simulink model "TECMD_OptimisationTemplate"  (R2021a)
settings: Solver=daessc  StartTime=0.0  StopTime=7192.4000005722046  FixedStep=1  MaxStep=1  RelTol=1e-3  AbsTol=1e-3
libraries: fl_lib x7, nesl_utility x7, BatteryLibrary_lib x1
settings Model: Creator=widana_d  LastModifiedBy=widana_d
settings SolverCC: AutoScaleAbsTol=off  AlgebraicLoopSolver=TrustRegion
settings DataIOCC: ExternalInput=currData  LoadExternalInput=on  SaveState=on  ReturnWorkspaceOutputsName=SDOSimTest_Log
settings DebuggingCC: SymbolicDimsDataTypeCodeGenerationDiagnostic=none  SFMachineParentedDataDiag=warning
settings SFSimCC: CustomCodeUndefinedFunction=UseInterfaceOnly
settings SimscapeCC: SimscapeLogType=all  SimscapeLogSimulationStatistics=on  SimscapeLogDataHistory=10000

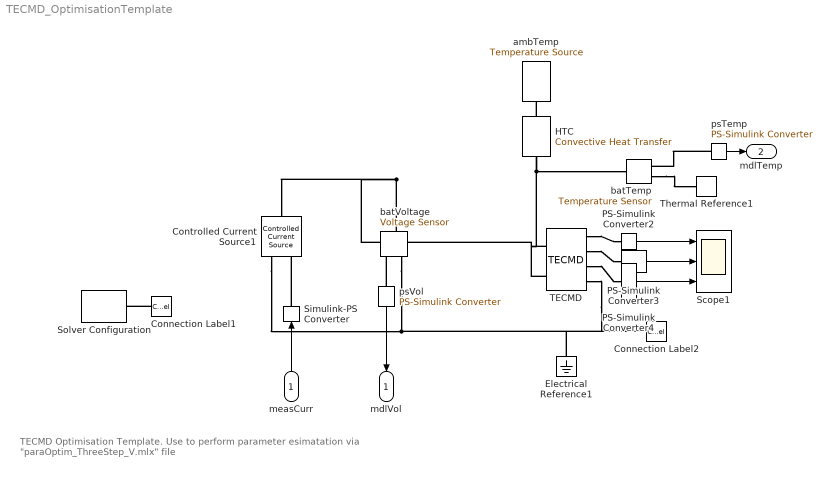
== system TECMD_OptimisationTemplate ==
  note: TECMD Optimisation Template.
      | Use to perform parameter esimatation via "paraOptim_ThreeStep_V.mlx" file
  measCurr : Inport
  Connection Label1 : ConnectionLabel  Label=solver
  Connection Label2 : ConnectionLabel  Label=solver
  Controlled Current Source1 : fl_lib/Electrical/Electrical Sources/Controlled Current Source
  Electrical Reference1 : fl_lib/Electrical/Electrical Elements/Electrical Reference
  HTC : fl_lib/Thermal/Thermal Elements/Convective Heat Transfer  area=cellArea m^2  heat_tr_coeff=h W/(m^2 * K)  T_specify=off  T_priority=None  T=0 K  T_nominal_specify=off  T_nominal_unit=K  T_nominal_value=1  Q_specify=off  Q_priority=None  Q=0 W  Q_nominal_specify=off  Q_nominal_unit=W  Q_nominal_value=1
  PS-Simulink Converter2 : nesl_utility/PS-Simulink Converter  PhysicalDomain=network_engine_domain  SubClassName=ps_output  LeftPortType=input  RightPortType=output  PseudoPeriodic=off  Frequencies=[]  Unit=inherit  AffineConversion=off
      settings: SourceProductBaseCode=PW,SS
  PS-Simulink Converter3 : nesl_utility/PS-Simulink Converter  PhysicalDomain=network_engine_domain  SubClassName=ps_output  LeftPortType=input  RightPortType=output  PseudoPeriodic=off  Frequencies=[]  Unit=inherit  AffineConversion=off
      settings: SourceProductBaseCode=PW,SS
  PS-Simulink Converter4 : nesl_utility/PS-Simulink Converter  PhysicalDomain=network_engine_domain  SubClassName=ps_output  LeftPortType=input  RightPortType=output  PseudoPeriodic=off  Frequencies=[]  Unit=inherit  AffineConversion=off
      settings: SourceProductBaseCode=PW,SS
  Scope1 : Scope  NumInputPorts=3
  Simulink-PS Converter : nesl_utility/Simulink-PS Converter  PhysicalDomain=network_engine_domain  SubClassName=ps_input  LeftPortType=input  RightPortType=output  PseudoPeriodic=off  Frequencies=[]  NoiseDistribution=none  NoiseParameters=[]  Unit=1  AffineConversion=off  FilteringAndDerivatives=provide  SimscapeFilterOrder=1  InputFilterTimeConstant=0.001  UdotUserProvided=0
      settings: SourceProductBaseCode=PW,SS
  Solver Configuration : nesl_utility/Solver Configuration  PhysicalDomain=network_engine_domain  SubClassName=solver  LeftPortType=input  RightPortType=generic  Tones=[]  Harmonics=[]  SimulateNoise=off  Profile=off  UseLocalSampling=off  EnableSwitchedLinearOptims=on  FrequencyDomain=off  UseCCode=off  RelTol=0.001  AbsTol=1e-06  MinStep=1e-09  ToWorkspace=off  RevertToSquareIcSolve=off  NumHomotopyIterations=100  PhasorMode=off  PhasorModeNumHarmonics=1  DoDC=off  ResidualTolerance=1e-09  UseLocalSolver=off  LocalSolverChoice=NE_BACKWARD_EULER_ADVANCER  LocalSolverSampleTime=0.001  DoFixedCost=off  MaxNonlinIter=3  MaxModeIter=2  ComputeImpulses=off  ImpulseIterations=2  LinearAlgebra=auto  EquationFormulation=NE_TIME_EF  DelaysMemoryBudget=1024  AutomaticFiltering=on  FilteringTimeConstant=0.001  PartitionStorageMethod=AS_NEEDED  PartitionMemoryBudget=1024  PartitionMethod=ROBUST
      settings: SourceProductName=Utilities
  TECMD : BatteryLibrary_lib/Models/TECMD  RoRef=RoRef Ohm  RpRef=RpRef Ohm  TaupRef=TaupRef s  TauRef=TauRef s  Cn=Cn hr*A  z0=z0  Cp=Cp J/K  Tref=Tref K  Ea_Ro=Ea_Ro kJ/mol  Ea_Rp=Ea_Rp kJ/mol  Ea_Taup=Ea_Taup kJ/mol  Ea_Tau=Ea_Tau kJ/mol  T0=T0 K  refSoC=[0 : 100]' / 100  refOCV=[2.8593, 2.9274, 2.9956, 3.061969, 3.1232121621911, 3.15470394885229, 3.18512081795661, 3.21447466451004, 3.23983418251859, 3.25947590964635, 3.27879990917066, 3.29791977833839, 3.31626752560394, 3.33307563518842, 3.34970466285667, 3.36646662161759, 3.38398642592777, 3.39826374829121, 3.41202994917722, 3.4257108806197, 3.43855191633442, 3.45201772552158, 3.46575676444741, 3.47936243182409, 3.49084733247506, 3.50171432332238, 3.51269575981572, 3.52363960685895, 3.5336162322311, 3.54266659043136, 3.55146484401725, 3.56028882406785, 3.57078460389872, 3.58129525123674, 3.59144125445442, 3.60158725767211, 3.6115458412695, 3.62096628333315, 3.63026578569043, 3.63956528804771, 3.64823659910672, 3.65653982870753, 3.66499745309439, 3.67345507748124, 3.68147228638747, 3.68961276847631, 3.69798562783594, 3.70635848719557, 3.71487037672799, 3.72380783932121, 3.73289437418429, 3.74198090904738, 3.75102505534397, 3.76031929016191, 3.76983942070008, 3.77935955123825, 3.78884224697143, 3.79882047635899, 3.80921579355511, 3.81961111075122, 3.83069866787416, 3.84218843373057, 3.85281884527956, 3.86344925682856, 3.873689991993, 3.8823694410751, 3.89044668294659, 3.89852392481808, 3.90617127176311, 3.91300386552967, 3.92012910853992, 3.92725435155017, 3.93469242351412, 3.94356346975952, 3.95323912490892, 3.96292857788519, 3.97285467951706, 3.98401645839863, 3.99554115817453, 4.00707749140522, 4.01845667704757, 4.02883766722974, 4.03842441517684, 4.0479611723355, 4.05712383581582, 4.06318824260145, 4.06769338009974, 4.07204669321773, 4.07628315129213, 4.07916567025178, 4.08185911816602, 4.08453654876338, 4.08729968783335, 4.09159374907186, 4.09693239670873, 4.10245989642775, 4.10817746663332, 4.12035945779669, 4.13522550585792, 4.15071368295431, 4.1662018600507]' V
      settings: InternalSimscapePortConfiguration="{\"Bottom\":[{\"id\":\"n\",\"label\":\"-\",\"type\":\"foundation.electrical.electrical\"}],\"Left\":[{\"id\":\"Hi\",\"label\":\"H\",\"type\":\"foundation.thermal.thermal\"}],\"Right\":[{\"id\":\"eta\",\"label\":\"Losses\",\"type\":\"output\"},{\"id\":\"OCV\",\"label\":\"OCV\",\"type\":\"output\"},{\"id\":\"zbar\",\"label\":\"SoC\",\"type\":\"output\"}],\"Top\":[{\"id\":\"p\",\"label\":\"+\",\"type\":\"foundation.electrical.electrical\"}]}"
  Thermal Reference1 : fl_lib/Thermal/Thermal Elements/Thermal Reference
  ambTemp : fl_lib/Thermal/Thermal Sources/Temperature Source  temperature=ambTemp K
  batTemp : fl_lib/Thermal/Thermal Sensors/Temperature Sensor
  batVoltage : fl_lib/Electrical/Electrical Sensors/Voltage Sensor
  psTemp : nesl_utility/PS-Simulink Converter  PhysicalDomain=network_engine_domain  SubClassName=ps_output  LeftPortType=input  RightPortType=output  PseudoPeriodic=off  Frequencies=[]  Unit=inherit  AffineConversion=off
      settings: SourceProductName=Utilities
  psVol : nesl_utility/PS-Simulink Converter  PhysicalDomain=network_engine_domain  SubClassName=ps_output  LeftPortType=input  RightPortType=output  PseudoPeriodic=off  Frequencies=[]  Unit=inherit  AffineConversion=off
      settings: SourceProductName=Utilities
  mdlVol : Outport
  mdlTemp : Outport  Port=2
  wires:
  measCurr/1 -> Simulink-PS Converter/1
  psTemp/1 -> mdlTemp/1
  psVol/1 -> mdlVol/1
  PS-Simulink Converter3/1 -> Scope1/2
  PS-Simulink Converter4/1 -> Scope1/3
  PS-Simulink Converter2/1 -> Scope1/1
  connections:
  batVoltage/LConn1 -- TECMD/LConn2 -- Controlled Current Source1/LConn1
  HTC/RConn1 -- ambTemp/LConn1
  HTC/LConn1 -- TECMD/LConn1 -- batTemp/LConn1
  batTemp/RConn1 -- Thermal Reference1/LConn1
  psVol/LConn1 -- batVoltage/RConn1
  psTemp/LConn1 -- batTemp/RConn2
  Connection Label1/LConn1 -- Solver Configuration/RConn1
  batVoltage/RConn2 -- Electrical Reference1/LConn1 -- Connection Label2/LConn1 -- TECMD/RConn4 -- Controlled Current Source1/RConn2
  Simulink-PS Converter/RConn1 -- Controlled Current Source1/RConn1
  TECMD/RConn1 -- PS-Simulink Converter2/LConn1
  TECMD/RConn3 -- PS-Simulink Converter4/LConn1
  TECMD/RConn2 -- PS-Simulink Converter3/LConn1
